simulink model "out_sub_PMSM_Base_MiL_controller"  (R2014a)
settings: Solver=FixedStepDiscrete  SolverMode=SingleTasking  StartTime=0.0  StopTime=1  FixedStep=1e-5  RelTol=1e-3
PreLoadFcn:
  | param_PMSM_Base
  | load('param_PMSM_Base.m');
undefined symbols (not defined in the file): ECU_MOTOR
libraries: simulink x1
settings Model: CovSFcnEnable=on  BufferReuse=off  Creator=Administrator  LastModifiedBy=yoshi12
settings DataIOCC: SignalLoggingSaveFormat=ModelDataLogs
settings OptimizationCC: ExpressionDepthLimit=2147483647  InitFltsAndDblsToZero=on  OptimizeModelRefInitCode=on  LifeSpan=1  SimCompilerOptimization=off
settings DebuggingCC: UnderspecifiedInitializationDetection=Classic  FcnCallInpInsideContextMsg=UseLocalSettings  FrameProcessingCompatibilityMsg=error  StateNameClashWarn=warning
settings SFSimCC: SimParseCustomCode=off
settings RTWCC: SystemTargetFile=ert.tlc  TemplateMakefile=ert_default_tmf  Description=Real-Time Workshop Embedded Coder (no auto configuration)  CreateSILPILBlock=SIL  RTWCompilerOptimization=off
settings CodeAppCC: IgnoreCustomStorageClasses=off  CustomSymbolStrType=$N$R$M  InternalIdentifier=Classic
settings ERTTargetCC: ParMdlRefBuildCompliant=on  CompOptLevelCompliant=on  ConcurrentExecutionCompliant=on  ERTFirstTimeCompliant=on  ModelStepFunctionPrototypeControlCompliant=on  CPPClassGenCompliant=on  ERTCustomFileTemplate=example_file_process.tlc

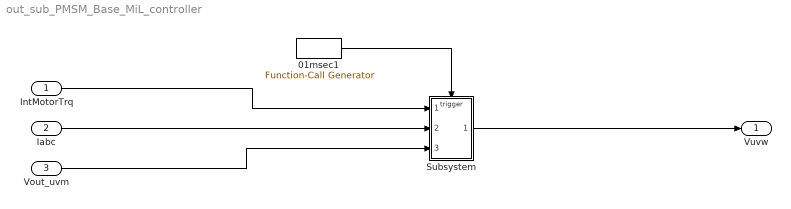
== system out_sub_PMSM_Base_MiL_controller ==
  IntMotorTrq : Inport
  Iabc : Inport  Port=2  PortDimensions=3
  Vout_uvm : Inport  Port=3  PortDimensions=3
  01msec1 : simulink/Ports & Subsystems/Function-Call Generator  sample_time=1e-4  numberOfIterations=1
  Subsystem : Subsystem
  Vuvw : Outport
  wires:
  IntMotorTrq/1 -> Subsystem/1(In1)
  Iabc/1 -> Subsystem/2(In2)
  Vout_uvm/1 -> Subsystem/3(In3)
  Subsystem/1(Vuvw) -> Vuvw/1
  01msec1/1 -> Subsystem/Trigger

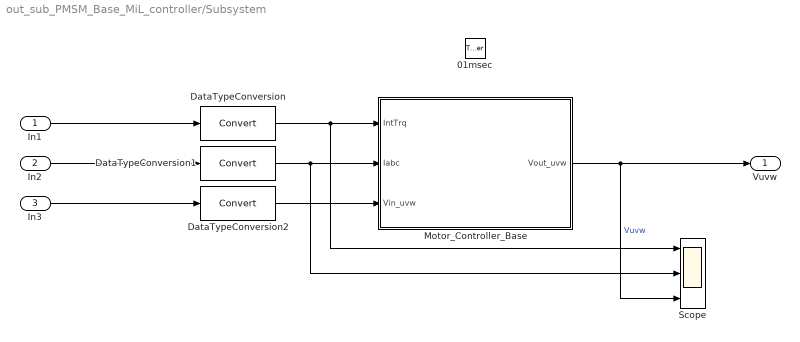
== system out_sub_PMSM_Base_MiL_controller/Subsystem ==
  In1 : Inport
  In2 : Inport  Port=2
  In3 : Inport  Port=3
  01msec : TriggerPort  TriggerType=function-call
  DataTypeConversion : DataTypeConversion
  DataTypeConversion1 : DataTypeConversion
  DataTypeConversion2 : DataTypeConversion
  Motor_Controller_Base : Subsystem  TreatAsAtomicUnit=on  mask{Phase_Idq=ECU_MOTOR.Phase_Idq, wc=ECU_MOTOR.wc, kp_d=ECU_MOTOR.kp_d, kp_q=ECU_MOTOR.kp_q, Ti_d=ECU_MOTOR.Ti_d, Ti_q=ECU_MOTOR.Ti_q, wsc=ECU_MOTOR.wsc, wpi=ECU_MOTOR.wpi, kp_v=ECU_MOTOR.kp_v, ki_v=ECU_MOTOR.ki_v, obs_onoff=ECU_MOTOR.obs_onoff, Tff=ECU_MOTOR.Tff, ff=ECU_MOTOR.ff, Phase_Loadtorque=ECU_MOTOR.Phase_Loadtorque, alpha_obs=ECU_MOTOR.alpha_obs, k1=ECU_MOTOR.k1, k2=ECU_MOTOR.k2, k3=ECU_MOTOR.k3, I=ECU_MOTOR.I, J=ECU_MOTOR.J, O=ECU_MOTOR.O, B1=ECU_MOTOR.B1, R=ECU_MOTOR.R, p=ECU_MOTOR.p, Ld=ECU_MOTOR.Ld, Lq=ECU_MOTOR.Lq, Rnt=ECU_MOTOR.Rnt, Ts=ECU_MOTOR.Ts, VDC=ECU_MOTOR.VDC, f_carrier=ECU_MOTOR.f_carrier, dvsw=ECU_MOTOR.dvsw}
      mask prompts: I ".I"
  Scope : Scope  NumInputPorts=3
      settings: YMin=-5~-5~-5  YMax=5~5~5  SaveName=MotorCtrlInOutData1
  Vuvw : Outport
  wires:
  In1/1 -> DataTypeConversion/1
  Motor_Controller_Base/1(Vout_uvw) -> Vuvw/1, Scope/3  "Vuvw"
  In2/1 -> DataTypeConversion1/1
  DataTypeConversion/1 -> Scope/1, Motor_Controller_Base/1(IntTrq)
  DataTypeConversion1/1 -> Scope/2, Motor_Controller_Base/2(Iabc)
  DataTypeConversion2/1 -> Motor_Controller_Base/3(Vin_uvw)
  In3/1 -> DataTypeConversion2/1

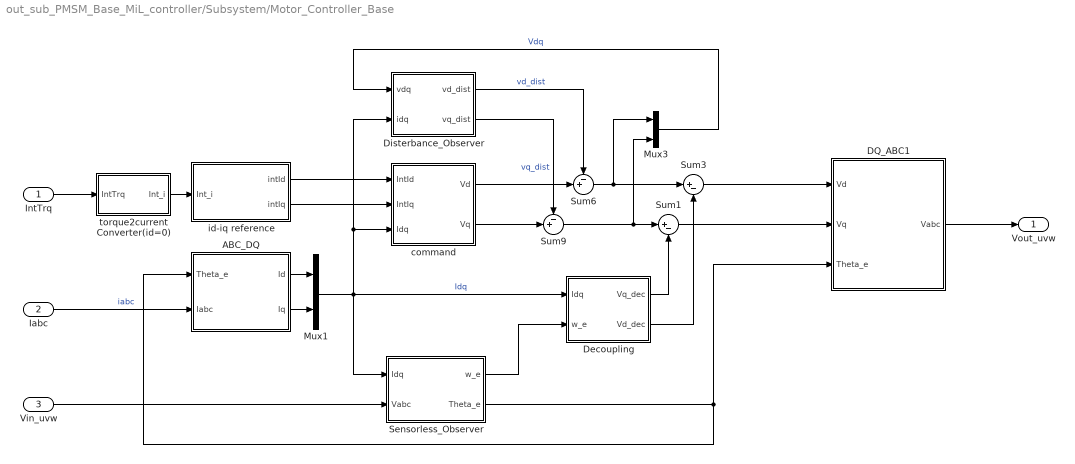
== system out_sub_PMSM_Base_MiL_controller/Subsystem/Motor_Controller_Base ==
  IntTrq : Inport
  Iabc : Inport  Port=2
  Vin_uvw : Inport  Port=3
  ABC_DQ : Subsystem
      mask Display: disp('abc-dq')
  DQ_ABC1 : Subsystem
      mask Display: disp('dq-abc')
  Decoupling : Subsystem
  Disterbance_Observer : Subsystem
  Mux1 : Mux  Inputs=2
  Mux3 : Mux  Inputs=2
  Sensorless_Observer : Subsystem
  Sum1 : Sum  Inputs=|+-
  Sum3 : Sum  Inputs=|+-
  Sum6 : Sum  Inputs=-+|
  Sum9 : Sum  Inputs=-+|
  command : Subsystem
  id-iq reference : Subsystem
  torque2current Converter(id=0) : Subsystem
  Vout_uvw : Outport
  wires:
  IntTrq/1 -> torque2current Converter(id=0)/1(IntTrq)
  id-iq reference/1(intId) -> command/1(IntId)
  id-iq reference/2(intIq) -> command/2(IntIq)
  DQ_ABC1/1(Vabc) -> Vout_uvw/1
  Iabc/1 -> ABC_DQ/2(Iabc)  "iabc"
  Sum3/1 -> DQ_ABC1/1(Vd)
  command/2(Vq) -> Sum9/2
  Sum1/1 -> DQ_ABC1/2(Vq)
  command/1(Vd) -> Sum6/2
  ABC_DQ/1(Id) -> Mux1/1
  ABC_DQ/2(Iq) -> Mux1/2
  Mux1/1 -> Disterbance_Observer/2(idq), command/3(Idq), Decoupling/1(Idq), Sensorless_Observer/1(Idq)  "Idq"
  Decoupling/2(Vd_dec) -> Sum3/2
  Decoupling/1(Vq_dec) -> Sum1/2
  torque2current Converter(id=0)/1(Int_i) -> id-iq reference/1(Int_i)
  Mux3/1 -> Disterbance_Observer/1(vdq)  "Vdq"
  Sum6/1 -> Mux3/1, Sum3/1
  Sum9/1 -> Sum1/1, Mux3/2
  Disterbance_Observer/2(vq_dist) -> Sum9/1  "vq_dist"
  Disterbance_Observer/1(vd_dist) -> Sum6/1  "vd_dist"
  Sensorless_Observer/1(w_e) -> Decoupling/2(w_e)
  Vin_uvw/1 -> Sensorless_Observer/2(Vabc)
  Sensorless_Observer/2(Theta_e) -> DQ_ABC1/3(Theta_e), ABC_DQ/1(Theta_e)

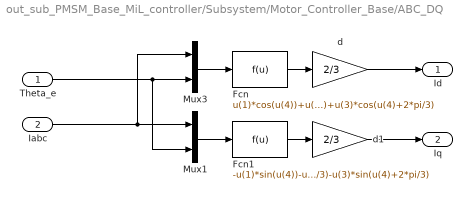
== system out_sub_PMSM_Base_MiL_controller/Subsystem/Motor_Controller_Base/ABC_DQ ==
  Theta_e : Inport
  Iabc : Inport  Port=2
  Fcn : Fcn  Expr=u(1)*cos(u(4))+u(2)*cos(u(4)-2*pi/3)+u(3)*cos(u(4)+2*pi/3)
  Fcn1 : Fcn  Expr=-u(1)*sin(u(4))-u(2)*sin(u(4)-2*pi/3)-u(3)*sin(u(4)+2*pi/3)
  Mux1 : Mux  Inputs=2
  Mux3 : Mux  Inputs=2
  d : Gain  Gain=2/3  OutDataTypeStr=Inherit: Same as input  ParamDataTypeStr=Inherit: Same as input
  d1 : Gain  Gain=2/3  OutDataTypeStr=Inherit: Same as input  ParamDataTypeStr=Inherit: Same as input
  Id : Outport  InitialOutput=0
  Iq : Outport  Port=2  InitialOutput=0
  wires:
  Theta_e/1 -> Mux3/2, Mux1/2
  Mux3/1 -> Fcn/1
  Fcn/1 -> d/1
  Mux1/1 -> Fcn1/1
  Fcn1/1 -> d1/1
  Iabc/1 -> Mux1/1, Mux3/1
  d/1 -> Id/1
  d1/1 -> Iq/1

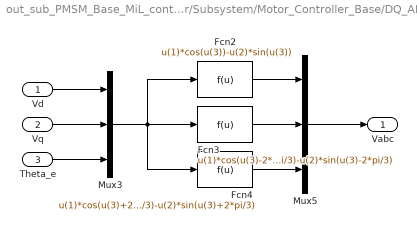
== system out_sub_PMSM_Base_MiL_controller/Subsystem/Motor_Controller_Base/DQ_ABC1 ==
  Vd : Inport
  Vq : Inport  Port=2
  Theta_e : Inport  Port=3
  Fcn2 : Fcn  Expr=u(1)*cos(u(3))-u(2)*sin(u(3))
  Fcn3 : Fcn  Expr=u(1)*cos(u(3)-2*pi/3)-u(2)*sin(u(3)-2*pi/3)
  Fcn4 : Fcn  Expr=u(1)*cos(u(3)+2*pi/3)-u(2)*sin(u(3)+2*pi/3)
  Mux3 : Mux  Inputs=3
  Mux5 : Mux  Inputs=3
  Vabc : Outport  InitialOutput=0
  wires:
  Fcn2/1 -> Mux5/1
  Mux5/1 -> Vabc/1
  Fcn3/1 -> Mux5/2
  Fcn4/1 -> Mux5/3
  Vd/1 -> Mux3/1
  Vq/1 -> Mux3/2
  Theta_e/1 -> Mux3/3
  Mux3/1 -> Fcn3/1, Fcn2/1, Fcn4/1

== system out_sub_PMSM_Base_MiL_controller/Subsystem/Motor_Controller_Base/Decoupling ==
  Idq : Inport
  w_e : Inport  Port=2
  Mux2 : Mux  Inputs=2
  _wLdid_wRnt : Fcn  Expr=-u(1)*Ld*u(2)-u(1)*Rnt
  wLqiq : Fcn  Expr=u(1)*Lq*u(3)
  Vq_dec : Outport
  Vd_dec : Outport  Port=2
  wires:
  Mux2/1 -> wLqiq/1, _wLdid_wRnt/1
  Idq/1 -> Mux2/2
  _wLdid_wRnt/1 -> Vq_dec/1
  w_e/1 -> Mux2/1
  wLqiq/1 -> Vd_dec/1

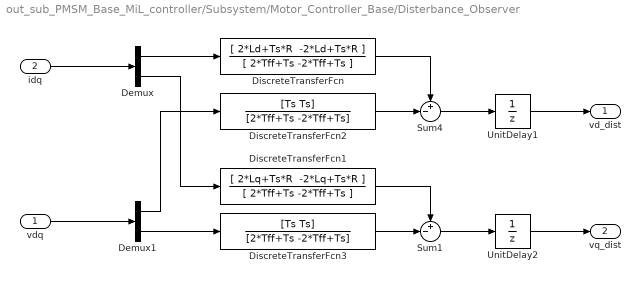
== system out_sub_PMSM_Base_MiL_controller/Subsystem/Motor_Controller_Base/Disterbance_Observer ==
  vdq : Inport
  idq : Inport  Port=2
  Demux : Demux  Outputs=2
  Demux1 : Demux  Outputs=2
  DiscreteTransferFcn : DiscreteTransferFcn  Numerator="[ 2*Ld+Ts*R  -2*Ld+Ts*R ]"  Denominator=[ 2*Tff+Ts -2*Tff+Ts ]
  DiscreteTransferFcn1 : DiscreteTransferFcn  Numerator="[ 2*Lq+Ts*R  -2*Lq+Ts*R ]"  Denominator=[ 2*Tff+Ts -2*Tff+Ts ]
  DiscreteTransferFcn2 : DiscreteTransferFcn  Numerator=[Ts Ts]  Denominator=[2*Tff+Ts -2*Tff+Ts]
  DiscreteTransferFcn3 : DiscreteTransferFcn  Numerator=[Ts Ts]  Denominator=[2*Tff+Ts -2*Tff+Ts]
  Sum1 : Sum  Inputs=+-|
  Sum4 : Sum  Inputs=+-|
  UnitDelay1 : UnitDelay  SampleTime=-1
  UnitDelay2 : UnitDelay  SampleTime=-1
  vd_dist : Outport
  vq_dist : Outport  Port=2
  wires:
  Demux1/1 -> DiscreteTransferFcn2/1
  Sum4/1 -> UnitDelay1/1
  Demux1/2 -> DiscreteTransferFcn3/1
  Demux/2 -> DiscreteTransferFcn1/1
  DiscreteTransferFcn3/1 -> Sum1/2
  Sum1/1 -> UnitDelay2/1
  Demux/1 -> DiscreteTransferFcn/1
  idq/1 -> Demux/1
  vdq/1 -> Demux1/1
  DiscreteTransferFcn/1 -> Sum4/1
  DiscreteTransferFcn1/1 -> Sum1/1
  UnitDelay1/1 -> vd_dist/1
  UnitDelay2/1 -> vq_dist/1
  DiscreteTransferFcn2/1 -> Sum4/2

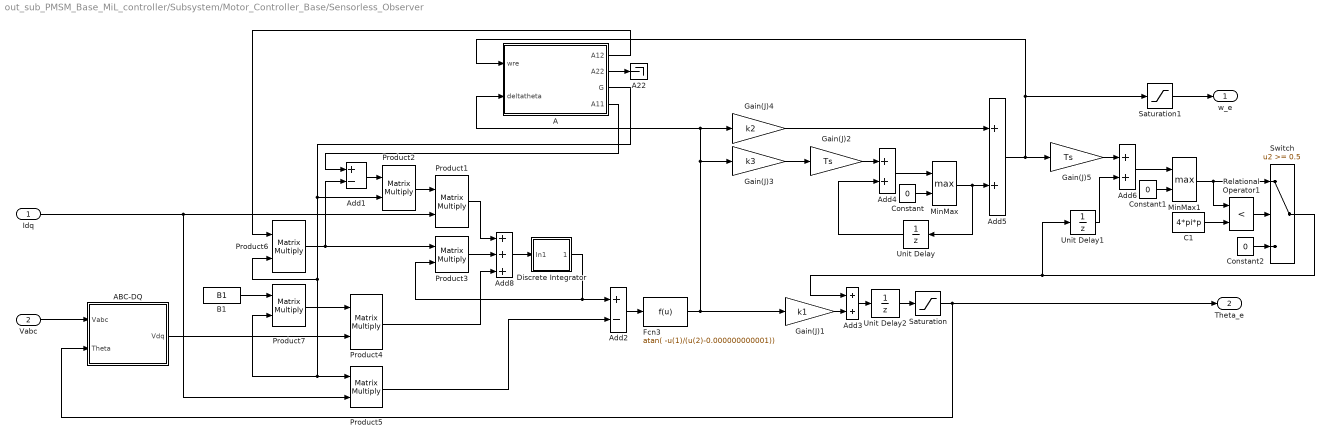
== system out_sub_PMSM_Base_MiL_controller/Subsystem/Motor_Controller_Base/Sensorless_Observer ==
  Idq : Inport
  Vabc : Inport  Port=2
  A : Subsystem
  A22 : Terminator
  ABC-DQ : Subsystem
      mask Display: disp('abc-dq')
  Add1 : Sum  Inputs=+-
  Add2 : Sum  Inputs=+-
  Add{3..6} (4 alike) : Sum
  Add8 : Sum  Inputs=+++
  B1 : Constant  Value=B1
  C1 : Constant  Value=4*pi*p
  Constant : Constant  Value=0
  Constant1 : Constant  Value=0
  Constant2 : Constant  Value=0
  Discrete Integrator : Subsystem
  Fcn3 : Fcn  Expr=atan( -u(1)/(u(2)-0.000000000001))
  Gain(J)1 : Gain  Gain=k1  OutDataTypeStr=Inherit: Same as input  ParamDataTypeStr=Inherit: Same as input
  Gain(J)2 : Gain  Gain=Ts  OutDataTypeStr=Inherit: Same as input  ParamDataTypeStr=Inherit: Same as input
  Gain(J)3 : Gain  Gain=k3  OutDataTypeStr=Inherit: Same as input  ParamDataTypeStr=Inherit: Same as input
  Gain(J)4 : Gain  Gain=k2  OutDataTypeStr=Inherit: Same as input  ParamDataTypeStr=Inherit: Same as input
  Gain(J)5 : Gain  Gain=Ts  OutDataTypeStr=Inherit: Same as input  ParamDataTypeStr=Inherit: Same as input
  MinMax : MinMax  Function=max  Inputs=2
  MinMax1 : MinMax  Function=max  Inputs=2
  Product{1..7} (7 alike) : Product  Multiplication=Matrix(*)  OutDataTypeStr=Inherit: Same as first input
  Relational Operator1 : RelationalOperator  Operator=<  OutDataTypeStr=boolean
  Saturation : Saturate  UpperLimit=1000000000  LowerLimit=0
  Saturation1 : Saturate  UpperLimit=inf  LowerLimit=0
  Switch : Switch  Threshold=0.5
  Unit Delay : UnitDelay  SampleTime=-1
  Unit Delay1 : UnitDelay  SampleTime=-1
  Unit Delay2 : UnitDelay  SampleTime=-1
  w_e : Outport
  Theta_e : Outport  Port=2
  wires:
  Discrete Integrator/1(Out1) -> Add2/1, Product3/2
  A/1(A12) -> Product6/1
  A/4(A11) -> Add1/1
  Gain(J)3/1 -> Gain(J)2/1
  Gain(J)4/1 -> Add5/1
  Add5/1 -> Gain(J)5/1, A/1(wre), Saturation1/1
  Add8/1 -> Discrete Integrator/1(In1)
  Product3/1 -> Add8/2
  Fcn3/1 -> Gain(J)1/1, A/2(deltatheta), Gain(J)4/1, Gain(J)3/1
  Product6/1 -> Product3/1, Add1/2
  A/3(G) -> Product5/1, Product7/2, Product6/2, Product2/2
  ABC-DQ/1(Vdq) -> Product4/2
  B1/1 -> Product7/1
  Product7/1 -> Product4/1
  Product4/1 -> Add8/3
  Add1/1 -> Product2/1
  Product2/1 -> Product1/1
  Product1/1 -> Add8/1
  Product5/1 -> Add2/2
  Add2/1 -> Fcn3/1
  Gain(J)1/1 -> Add3/2
  Add3/1 -> Unit Delay2/1
  Unit Delay2/1 -> Saturation/1
  A/2(A22) -> A22/1
  Idq/1 -> Product1/2, Product5/2
  Vabc/1 -> ABC-DQ/1(Vabc)
  Saturation/1 -> Theta_e/1, ABC-DQ/2(Theta)
  Saturation1/1 -> w_e/1
  Constant/1 -> MinMax/2
  Unit Delay/1 -> Add4/2
  Add4/1 -> MinMax/1
  MinMax/1 -> Unit Delay/1, Add5/2
  Gain(J)2/1 -> Add4/1
  Constant1/1 -> MinMax1/2
  MinMax1/1 -> Relational Operator1/1, Switch/1
  Add6/1 -> MinMax1/1
  C1/1 -> Relational Operator1/2
  Gain(J)5/1 -> Add6/1
  Relational Operator1/1 -> Switch/2
  Constant2/1 -> Switch/3
  Switch/1 -> Add3/1, Unit Delay1/1
  Unit Delay1/1 -> Add6/2

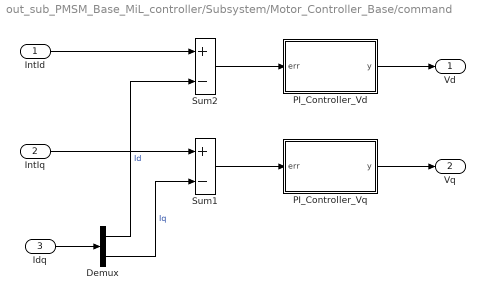
== system out_sub_PMSM_Base_MiL_controller/Subsystem/Motor_Controller_Base/command ==
  IntId : Inport
  IntIq : Inport  Port=2
  Idq : Inport  Port=3
  Demux : Demux  Outputs=2
  PI_Controller_Vd : Subsystem
  PI_Controller_Vq : Subsystem
  Sum1 : Sum  Inputs=+-  InputSameDT=on  OutDataTypeStr=Inherit: Same as first input
  Sum2 : Sum  Inputs=+-  InputSameDT=on  OutDataTypeStr=Inherit: Same as first input
  Vd : Outport
  Vq : Outport  Port=2
  wires:
  IntId/1 -> Sum2/1
  PI_Controller_Vd/1(y) -> Vd/1
  Sum2/1 -> PI_Controller_Vd/1(err)
  Idq/1 -> Demux/1
  PI_Controller_Vq/1(y) -> Vq/1
  Sum1/1 -> PI_Controller_Vq/1(err)
  IntIq/1 -> Sum1/1
  Demux/1 -> Sum2/2  "Id"
  Demux/2 -> Sum1/2  "Iq"

== system out_sub_PMSM_Base_MiL_controller/Subsystem/Motor_Controller_Base/id-iq reference ==
  Int_i : Inport
  Constant : Constant  Value=0
  intId : Outport
  intIq : Outport  Port=2
  wires:
  Int_i/1 -> intIq/1
  Constant/1 -> intId/1

== system out_sub_PMSM_Base_MiL_controller/Subsystem/Motor_Controller_Base/torque2current Converter(id=0) ==
  note: Assuming, id=0 (ie. Phase_idq=pi/2)
  IntTrq : Inport
  Constant : Constant  Value=1.5
  Constant1 : Constant  Value=p
  Constant2 : Constant  Value=Rnt
  Product : Product  Inputs=*///  RndMeth=Zero
  Int_i : Outport
  wires:
  Product/1 -> Int_i/1
  IntTrq/1 -> Product/1
  Constant/1 -> Product/2
  Constant1/1 -> Product/3
  Constant2/1 -> Product/4

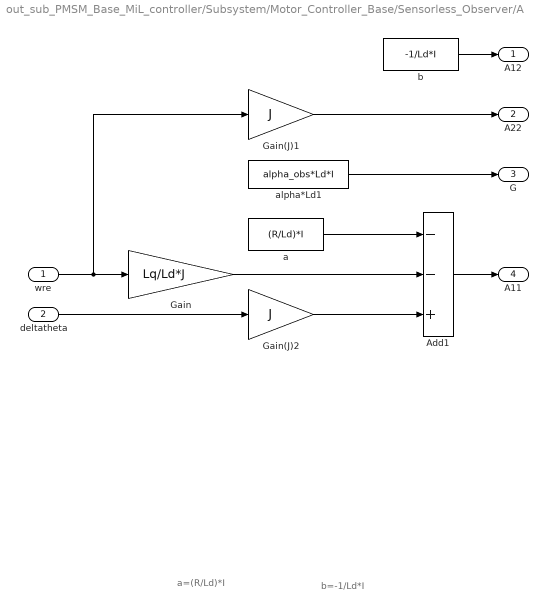
== system out_sub_PMSM_Base_MiL_controller/Subsystem/Motor_Controller_Base/Sensorless_Observer/A ==
  note: b=-1/Ld*I
  note: a=(R/Ld)*I
  wre : Inport
  deltatheta : Inport  Port=2
  Add1 : Sum  Inputs=--+
  Gain : Gain  Gain=Lq/Ld*J
  Gain(J)1 : Gain  Gain=J  OutDataTypeStr=Inherit: Same as input  ParamDataTypeStr=Inherit: Same as input
  Gain(J)2 : Gain  Gain=J  OutDataTypeStr=Inherit: Same as input  ParamDataTypeStr=Inherit: Same as input
  a : Constant  Value=(R/Ld)*I
  alpha*Ld1 : Constant  Value=alpha_obs*Ld*I
  b : Constant  Value=-1/Ld*I
  A12 : Outport
  A22 : Outport  Port=2
  G : Outport  Port=3
  A11 : Outport  Port=4
  wires:
  Gain(J)1/1 -> A22/1
  b/1 -> A12/1
  Add1/1 -> A11/1
  Gain/1 -> Add1/2
  a/1 -> Add1/1
  wre/1 -> Gain/1, Gain(J)1/1
  deltatheta/1 -> Gain(J)2/1
  alpha*Ld1/1 -> G/1
  Gain(J)2/1 -> Add1/3

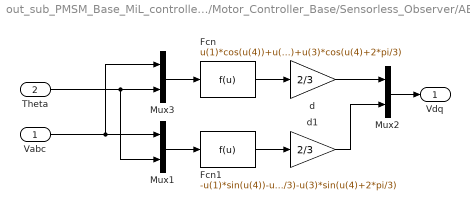
== system out_sub_PMSM_Base_MiL_controller/Subsystem/Motor_Controller_Base/Sensorless_Observer/ABC-DQ ==
  Vabc : Inport
  Theta : Inport  Port=2
  Fcn : Fcn  Expr=u(1)*cos(u(4))+u(2)*cos(u(4)-2*pi/3)+u(3)*cos(u(4)+2*pi/3)
  Fcn1 : Fcn  Expr=-u(1)*sin(u(4))-u(2)*sin(u(4)-2*pi/3)-u(3)*sin(u(4)+2*pi/3)
  Mux1 : Mux  Inputs=2
  Mux2 : Mux  Inputs=2
  Mux3 : Mux  Inputs=2
  d : Gain  Gain=2/3  OutDataTypeStr=Inherit: Same as input  ParamDataTypeStr=Inherit: Same as input
  d1 : Gain  Gain=2/3  OutDataTypeStr=Inherit: Same as input  ParamDataTypeStr=Inherit: Same as input
  Vdq : Outport  InitialOutput=0
  wires:
  d/1 -> Mux2/1
  Mux2/1 -> Vdq/1
  d1/1 -> Mux2/2
  Vabc/1 -> Mux3/1, Mux1/1
  Fcn1/1 -> d1/1
  Mux1/1 -> Fcn1/1
  Fcn/1 -> d/1
  Mux3/1 -> Fcn/1
  Theta/1 -> Mux1/2, Mux3/2

== system out_sub_PMSM_Base_MiL_controller/Subsystem/Motor_Controller_Base/Sensorless_Observer/Discrete Integrator ==
  In1 : Inport
  Add7 : Sum
  Gain(J)6 : Gain  Gain=Ts  OutDataTypeStr=Inherit: Same as input  ParamDataTypeStr=Inherit: Same as input
  Unit Delay3 : UnitDelay  SampleTime=-1
  Out1 : Outport
  wires:
  Gain(J)6/1 -> Add7/1
  In1/1 -> Gain(J)6/1
  Add7/1 -> Unit Delay3/1
  Unit Delay3/1 -> Out1/1, Add7/2

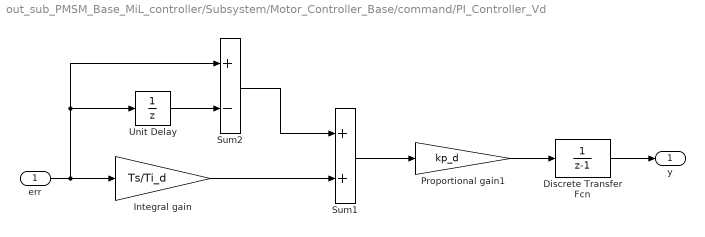
== system out_sub_PMSM_Base_MiL_controller/Subsystem/Motor_Controller_Base/command/PI_Controller_Vd ==
  err : Inport
  Discrete Transfer Fcn : DiscreteTransferFcn  Numerator=1  Denominator=[1 -1]
  Integral gain : Gain  Gain=Ts/Ti_d  OutDataTypeStr=Inherit: Same as input  ParamDataTypeStr=Inherit: Same as input
  Proportional gain1 : Gain  Gain=kp_d  OutDataTypeStr=Inherit: Same as input  ParamDataTypeStr=Inherit: Same as input
  Sum1 : Sum  InputSameDT=on  OutDataTypeStr=Inherit: Same as first input
  Sum2 : Sum  Inputs=+-  InputSameDT=on  OutDataTypeStr=Inherit: Same as first input
  Unit Delay : UnitDelay  SampleTime=-1
  y : Outport
  wires:
  err/1 -> Integral gain/1, Sum2/1, Unit Delay/1
  Sum1/1 -> Proportional gain1/1
  Integral gain/1 -> Sum1/2
  Proportional gain1/1 -> Discrete Transfer Fcn/1
  Unit Delay/1 -> Sum2/2
  Sum2/1 -> Sum1/1
  Discrete Transfer Fcn/1 -> y/1

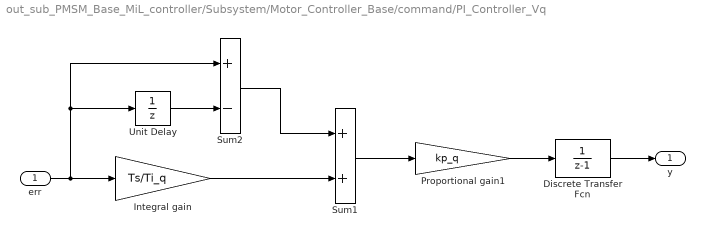
== system out_sub_PMSM_Base_MiL_controller/Subsystem/Motor_Controller_Base/command/PI_Controller_Vq ==
  err : Inport
  Discrete Transfer Fcn : DiscreteTransferFcn  Numerator=1  Denominator=[1 -1]
  Integral gain : Gain  Gain=Ts/Ti_q  OutDataTypeStr=Inherit: Same as input  ParamDataTypeStr=Inherit: Same as input
  Proportional gain1 : Gain  Gain=kp_q  OutDataTypeStr=Inherit: Same as input  ParamDataTypeStr=Inherit: Same as input
  Sum1 : Sum  InputSameDT=on  OutDataTypeStr=Inherit: Same as first input
  Sum2 : Sum  Inputs=+-  InputSameDT=on  OutDataTypeStr=Inherit: Same as first input
  Unit Delay : UnitDelay  SampleTime=-1
  y : Outport
  wires:
  Discrete Transfer Fcn/1 -> y/1
  Sum2/1 -> Sum1/1
  Unit Delay/1 -> Sum2/2
  Proportional gain1/1 -> Discrete Transfer Fcn/1
  Integral gain/1 -> Sum1/2
  Sum1/1 -> Proportional gain1/1
  err/1 -> Unit Delay/1, Sum2/1, Integral gain/1
